simulink model "chua_c_sim"  (R2022b)
settings: Solver=ode23t  StartTime=0.0  StopTime=Tfin  RelTol=1e-3
values from neighbouring files (symbols this model uses):
  ie = 1    [main_chua.m]
  K = place(A{ie},g,[-1,-2,-3])    [main_chua.m]
  x0 = randn(3,1)*0.2    [main_chua.m]
undefined symbols (not defined in the file or in its folder): fg_chua, xeq
settings Model: Creator=carlonovara  LastModifiedBy=Enf
settings SolverCC: AlgebraicLoopSolver=TrustRegion
settings DataIOCC: ReturnWorkspaceOutputs=off
settings DebuggingCC: UnconnectedInputMsg=warning  UnconnectedOutputMsg=warning  UnconnectedLineMsg=warning  SFMachineParentedDataDiag=warning  ArithmeticOperatorsInVariantConditions=warning
settings ModelReferenceCC: EnableRefExpFcnMdlSchedulingChecks=on
settings SFSimCC: SimUseLocalCustomCode=off  CustomCodeUndefinedFunction=UseInterfaceOnly
settings RTWCC: RTWUseLocalCustomCode=off
settings CodeAppCC: StateflowObjectComments=on

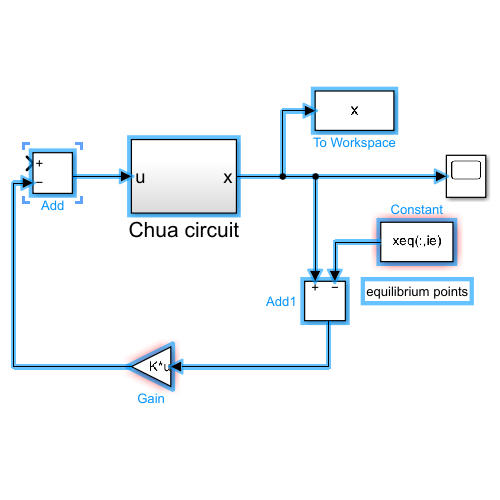
[thumbnail: Simulink's stored preview of the top-level diagram]
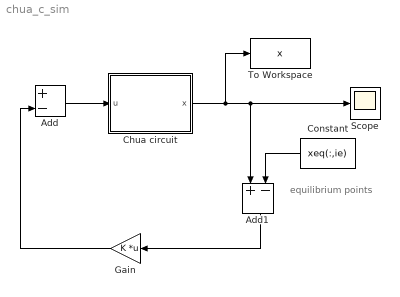
== system chua_c_sim ==
  note: equilibrium points
  Add : Sum  Inputs=+-
  Add1 : Sum  Inputs=+-
  Chua circuit : Subsystem
  Constant : Constant  Value=xeq(:,ie)
  Gain : Gain  Gain=K  Multiplication=Matrix(K*u)
  Scope : Scope
  To Workspace : ToWorkspace  VariableName=x  SampleTime=-1
  wires:
  Chua circuit/1(x) -> Scope/1, Add1/1, To Workspace/1
  Add/1 -> Chua circuit/1(u)
  Gain/1 -> Add/2
  Add1/1 -> Gain/1
  Constant/1 -> Add1/2

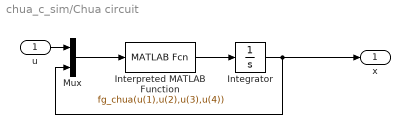
== system chua_c_sim/Chua circuit ==
  u : Inport
  Integrator : Integrator  InitialCondition=x0
  Interpreted MATLAB Function : MATLABFcn  MATLABFcn=fg_chua(u(1),u(2),u(3),u(4))  OutputDimensions=3
  Mux : Mux  Inputs=2
  x : Outport  VectorParamsAs1DForOutWhenUnconnected=off
  wires:
  u/1 -> Mux/1
  Interpreted MATLAB Function/1 -> Integrator/1
  Integrator/1 -> Mux/2, x/1
  Mux/1 -> Interpreted MATLAB Function/1
